simulink model "Electron_Energization_Index_v3"  (R2020a)
settings: Solver=ode45  StartTime=0.0  StopTime=100  RelTol=1e-3  EnableMultiTasking=on
values from neighbouring files (symbols this model uses):
  alpha_d = 4    [Electron_Energization_Index_v3_0_parameters.m]
  alpha_I = 1    [Electron_Energization_Index_v3_0_parameters.m]
  c3 = 2    [Electron_Energization_Index_v3_0_parameters.m]
  step_time = 5    [Electron_Energization_Index_v3_0_parameters.m]
  t_delay = 35    [Electron_Energization_Index_v3_0_parameters.m]    (also in windmi.m = -(250*6380)/mean(1.0*Vx))
  tau_loss = 15    [Electron_Energization_Index_v3_0_parameters.m]
settings Model: Creator=edmund  LastModifiedBy=pavit
settings SolverCC: ZeroCrossAlgorithm=Adaptive
settings DataIOCC: LimitDataPoints=on  SaveFormat=Array  ReturnWorkspaceOutputs=off
settings OptimizationCC: LifeSpan=inf
settings DebuggingCC: SFUnexpectedBacktrackingDiag=warning  SFNoUnconditionalDefaultTransitionDiag=warning  SFExecutionAtInitializationDiag=none  ArithmeticOperatorsInVariantConditions=warning
settings HardwareCC: ProdBitPerPointer=32  ProdBitPerSizeT=32  ProdBitPerPtrDiffT=32  ProdLargestAtomicFloat=None  ProdIntDivRoundTo=Undefined  ProdEndianess=Unspecified  ProdWordSize=32  ProdHWDeviceType=32-bit Generic
settings ModelReferenceCC: PropagateSignalLabelsOutOfModel=off
settings SFSimCC: SimUseLocalCustomCode=off  CustomCodeUndefinedFunction=UseInterfaceOnly
settings RTWCC: RTWUseLocalCustomCode=off
settings CodeAppCC: StateflowObjectComments=on
settings GRTTargetCC: TargetLangStandard=C89/C90 (ANSI)
settings ConfigComp: CovMetricSettings=dw  CovHtmlReporting=on  CovSaveCumulativeToWorkspaceVar=on  CovSaveSingleToWorkspaceVar=on  CovExternalEMLEnable=off  CovSFcnEnable=off

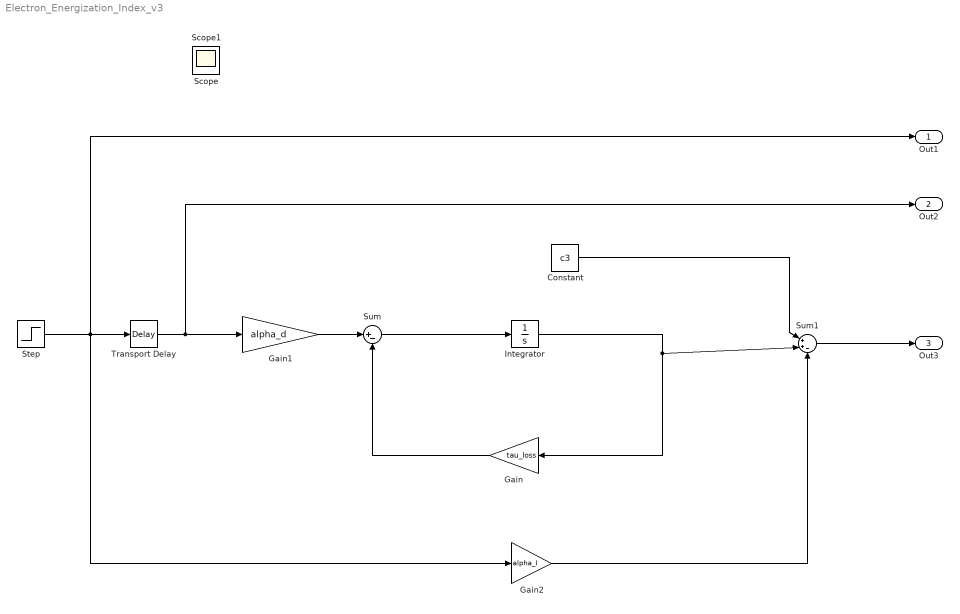
== system Electron_Energization_Index_v3 ==
  Constant : Constant  Value=c3
  Gain : Gain  Gain=tau_loss
  Gain1 : Gain  Gain=alpha_d
  Gain2 : Gain  Gain=alpha_I
  Integrator : Integrator
  Step : Step  Time=step_time  SampleTime=0.01
  Sum : Sum  Inputs=|+-
  Sum1 : Sum  Inputs=|++-
  Transport Delay : TransportDelay  DelayTime=t_delay
  Out1 : Outport
  Out2 : Outport  Port=2
  Out3 : Outport  Port=3
  Scope : Scope
  Scope1 : Scope
  wires:
  Integrator/1 -> Sum1/2, Gain/1
  Sum/1 -> Integrator/1
  Gain1/1 -> Sum/1
  Gain/1 -> Sum/2
  Constant/1 -> Sum1/1
  Step/1 -> Out1/1, Gain2/1, Transport Delay/1
  Transport Delay/1 -> Out2/1, Gain1/1
  Gain2/1 -> Sum1/3
  Sum1/1 -> Out3/1
